simulink model "dve_nadrze_nelinear"  (R2016a)
settings: Solver=VariableStepAuto  SolverMode=SingleTasking  StartTime=0.0  StopTime=t  RelTol=1e-3
undefined symbols (not defined in the file): c2, cp, dQ, g, h1condition, h2condition, S, S2, Sp, stepTime, U
settings Model: Creator=Filip Jašek  LastModifiedBy=Filip Jašek
settings DataIOCC: ReturnWorkspaceOutputs=on
settings DebuggingCC: SFUnexpectedBacktrackingDiag=error  SFNoUnconditionalDefaultTransitionDiag=error
settings SFSimCC: SimUseLocalCustomCode=on
settings RTWCC: RTWUseLocalCustomCode=on
settings GRTTargetCC: TargetLangStandard=C99 (ISO)
settings ConfigComp: CovMetricSettings=dwe  CovHtmlReporting=off  CovSaveCumulativeToWorkspaceVar=off  CovSaveSingleToWorkspaceVar=off  CovExternalEMLEnable=on

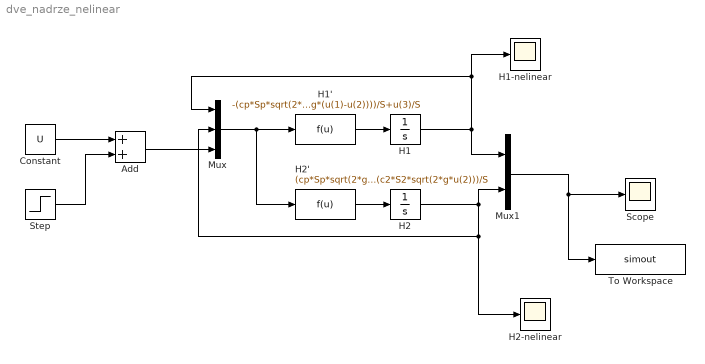
== system dve_nadrze_nelinear ==
  Add : Sum
  Constant : Constant  Value=U
  H1 : Integrator  InitialCondition=h1condition
  H1' : Fcn  Expr=-(cp*Sp*sqrt(2*g*(u(1)-u(2))))/S+u(3)/S
  H1-nelinear : Scope
  H2 : Integrator  InitialCondition=h2condition
  H2' : Fcn  Expr=(cp*Sp*sqrt(2*g*(u(1)-u(2))))/S-(c2*S2*sqrt(2*g*u(2)))/S
  H2-nelinear : Scope
  Mux : Mux  Inputs=3
  Mux1 : Mux  Inputs=2
  Scope : Scope
  Step : Step  Time=stepTime  After=dQ  SampleTime=0
  To Workspace : ToWorkspace  VariableName=simout  SaveFormat=Timeseries  SampleTime=-1
  wires:
  Mux/1 -> H2'/1, H1'/1
  H2/1 -> H2-nelinear/1, Mux/2, Mux1/2
  Mux1/1 -> To Workspace/1, Scope/1
  H2'/1 -> H2/1
  H1/1 -> H1-nelinear/1, Mux/1, Mux1/1
  H1'/1 -> H1/1
  Constant/1 -> Add/1
  Add/1 -> Mux/3
  Step/1 -> Add/2
